simulink model "GCU_Model"  (R2018a)
settings: Solver=FixedStepDiscrete  StartTime=0.0  StopTime=1000.0  FixedStep=0.001  RelTol=1e-3  EnableMultiTasking=on
undefined symbols (not defined in the file): sigbuilder_block
libraries: simulink x1
settings Model: PacingRate=0.063000  Creator=SIMONE  LastModifiedBy=SIMONE
settings SolverCC: AutoInsertRateTranBlk=on
settings OptimizationCC: DefaultParameterBehavior=Inlined  UseFloatMulNetSlope=on  InlineInvariantSignals=on  PassReuseOutputArgsAs=Individual arguments  ZeroExternalMemoryAtStartup=off  ZeroInternalMemoryAtStartup=off  NoFixptDivByZeroProtection=on  EfficientFloat2IntCast=on  LifeSpan=1  OptimizeBlockOrder=speed  DifferentSizesBufferReuse=on
settings DebuggingCC: ParameterTunabilityLossMsg=error
settings HardwareCC: ProdBitPerPointer=32  ProdBitPerSizeT=32  ProdBitPerPtrDiffT=32  ProdLargestAtomicInteger=Long  ProdLargestAtomicFloat=Double  ProdWordSize=32  ProdLongLongMode=on  ProdHWDeviceType=ARM Compatible->ARM Cortex
settings ModelReferenceCC: ModelReferenceNumInstancesAllowed=Single
settings SFSimCC: MATLABDynamicMemAlloc=off
settings RTWCC: SystemTargetFile=ert.tlc  TemplateMakefile=ert_default_tmf  GenerateReport=on  IncludeHyperlinkInReport=on  LaunchReport=on  GenerateTraceInfo=on  GenerateTraceReport=on  GenerateTraceReportSl=on  GenerateTraceReportSf=on  GenerateTraceReportEml=on  GenerateCodeMetricsReport=on
settings CodeAppCC: ForceParamTrailComments=on  IgnoreCustomStorageClasses=off  OperatorAnnotations=on  SimulinkDataObjDesc=on  SFDataObjDesc=on  InsertBlockDesc=on
settings ERTTargetCC: TargetLangStandard=C99 (ISO)  GenerateSampleERTMain=on  IncludeMdlTerminateFcn=off  CombineSignalStateStructs=on  SupportNonFinite=off  SupportComplex=off  PurelyIntegerCode=on  SupportContinuousTime=on  SupportNonInlinedSFcns=on  InlinedParameterPlacement=NonHierarchical  ERTCustomFileTemplate=example_file_process.tlc  ERTFilePackagingFormat=CompactWithDataFile

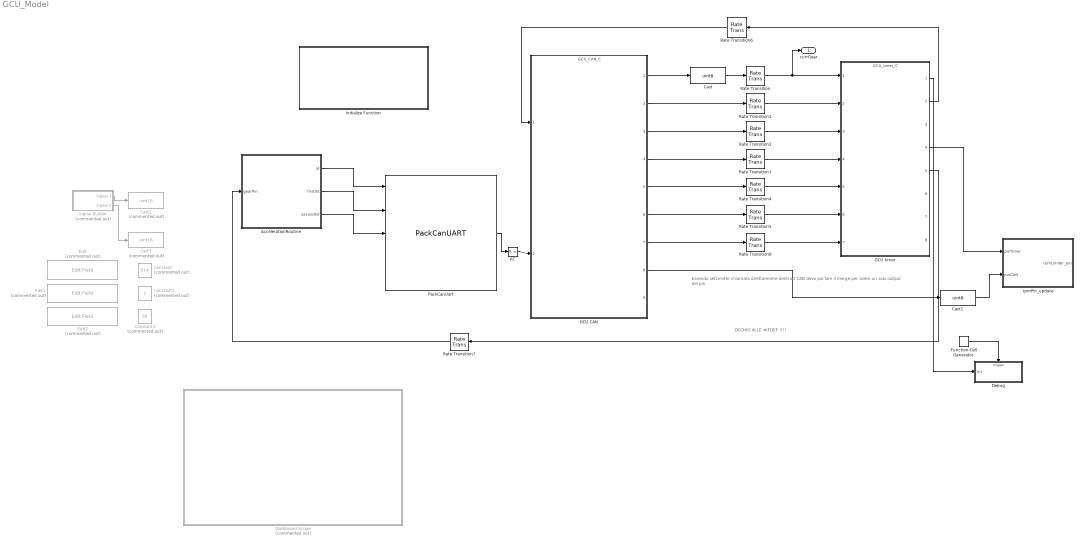
== system GCU_Model ==
  note: Essendo setLimiter chiamata direttamente dentro il CAN devo poi fare il merge
      | per avere un solo output del pin
  note: OCCHIO ALLE #IFDEF !!!!
  AccelerationRoutine : Stateflow chart  TreatAsAtomicUnit=on  SystemSampleTime=[0.01, 0.002]
  Cast : DataTypeConversion  OutDataTypeStr=uint8
  Cast1 : DataTypeConversion  OutDataTypeStr=uint8
  Cast2 : DataTypeConversion  Commented=on  OutDataTypeStr=uint16
  Cast3 : DataTypeConversion  Commented=on  OutDataTypeStr=uint16
  Constant : Constant  Commented=on  Value=514  OutDataTypeStr=uint16
  Constant2 : Constant  Commented=on  Value=2  OutDataTypeStr=uint16
  Constant3 : Constant  Commented=on  Value=30  OutDataTypeStr=uint16
  Dashboard Scope : Subsystem  Commented=on  DialogController=hmiCreateDDGDialog  IsWebBlock=on  mask(MWDashboardBlock){webBlockId=2eaf4557-9590-4f1a-91d6-635638ba46b2, webBlockType=sdiscope, ShowInitialText=on, HMISrcModelName=GCU_Model}
      mask prompts: webBlockId "WebBlock Id"; webBlockType "WebBlock Type"; HMISrcModelName "Source Model"
      mask help: SimulinkHMI:dialogs:HMIScopeDialogDesc
      mask Help: helpview([docroot '/mapfiles/simulink.map'], 'hmi_scope')
      mask Display:
      | if strcmp(get_param(bdroot(gcb),'BlockDiagramType'), 'library')
      |     image([(matlabroot) '/toolbox/simulink/hmi/icons/DashboardScope.png']);
      | end
  "Debug " : Subsystem  TreatAsAtomicUnit=on
  Edit : EditField  Commented=on  WebBlockId=100  LabelPosition=Hide  Alignment=Center
  Edit1 : EditField  Commented=on  WebBlockId=102  LabelPosition=Hide  Alignment=Center
  Edit2 : EditField  Commented=on  WebBlockId=104  LabelPosition=Hide  Alignment=Center
  Function-Call Generator : simulink/Ports & Subsystems/Function-Call Generator  sample_time=1  numberOfIterations=1
  GCU CAN : ModelReference  ModelNameDialog=GCU_CAN_C.slx  SimulationMode=Normal  ModelReferenceVersion=1.5
  GCU timer : ModelReference  ModelNameDialog=GCU_timer_C  SimulationMode=Normal  ModelReferenceVersion=1.9
  Initialize Function : Subsystem  TreatAsAtomicUnit=on
  PackCanUart : S-Function  FunctionName=PackCanUART  SFunctionDeploymentMode=off  EnableBusSupport=off
  RT : RateTransition  Deterministic=off  OutPortSampleTime=0.01
  Rate Transition{,1..8} (9 alike) : RateTransition  Deterministic=off
  Signal Builder : Subsystem  Tag=STV Subsys  Commented=on  LoadFcn=sigbuilder_block('load');  StartFcn=sigbuilder_block('start');  StopFcn=sigbuilder_block('stop');  ClipboardFcn=sigbuilder_block('clipboard');  mask(Sigbuilder block){tuvar=[0:10]}
      mask help: Simulink:masks:SigbuilderBlock_MD
      mask init:
      | if ~strcmp(get_param(bdroot(gcbh),'SimulationStatus'),'stopped') tuvar = sigbuilder_block('maskInit'); end
      settings: CopyFcn=sigbuilder_block('copy');  DeleteFcn=sigbuilder_block('delete');  ModelCloseFcn=sigbuilder_block('modelClose');  PreSaveFcn=sigbuilder_block('preSave');  PauseFcn=sigbuilder_block('pause');  ContinueFcn=sigbuilder_block('continue');  NameChangeFcn=sigbuilder_block('namechange');  OpenFcn=sigbuilder_block('open',[437.25 153 550.5 359.25 ]);  CloseFcn=sigbuilder_block('close');
      mask Display: plot(0, 0, 100, 100,[2, 2, 32, 32, 2], [68, 8, 8, 68, 68],[32, 2], [38, 38], [32, 19, 2],[53, 60, 44], [32, 17, 17, 2],[16, 16, 31, 31]);txt = getActiveGroup(gcbh);text(2, 100, txt,'verticalAlignment', 'top');
  rpmPin_update : Subsystem
  currGear : Outport
  wires:
  Signal Builder/2(Signal 2) -> Cast3/1
  Signal Builder/1(Signal 1) -> Cast2/1
  GCU CAN/1 -> Cast/1
  Rate Transition/1 -> GCU timer/1, currGear/1
  GCU CAN/2 -> Rate Transition1/1
  Rate Transition1/1 -> GCU timer/2
  GCU CAN/3 -> Rate Transition2/1
  Rate Transition2/1 -> GCU timer/3
  GCU CAN/4 -> Rate Transition3/1
  Rate Transition3/1 -> GCU timer/4
  GCU CAN/5 -> Rate Transition4/1
  Rate Transition4/1 -> GCU timer/5
  GCU CAN/6 -> Rate Transition5/1
  Rate Transition5/1 -> GCU timer/6
  GCU timer/2 -> Rate Transition6/1
  Rate Transition6/1 -> GCU CAN/1
  Cast/1 -> Rate Transition/1
  PackCanUart/1 -> RT/1
  GCU timer/5 -> Rate Transition7/1
  Rate Transition7/1 -> AccelerationRoutine/1(gearPin)
  GCU timer/4 -> rpmPin_update/1(pinTimer)
  GCU CAN/8 -> Cast1/1
  AccelerationRoutine/1(id) -> PackCanUart/1
  AccelerationRoutine/2(firstInt) -> PackCanUart/2
  AccelerationRoutine/3(secondInt) -> PackCanUart/3
  RT/1 -> GCU CAN/2
  GCU CAN/7 -> Rate Transition8/1
  Rate Transition8/1 -> GCU timer/7
  Cast1/1 -> rpmPin_update/2(pinCAN)
  Function-Call Generator/1 -> "Debug "/Trigger
  GCU timer/1 -> "Debug "/1(In1)

== system GCU_Model/Dashboard Scope ==

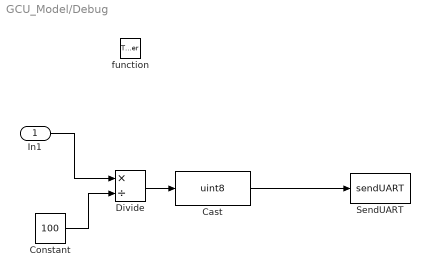
== system GCU_Model/Debug  ==
  In1 : Inport
  function : TriggerPort  TriggerType=function-call  VariantControl=Variant
  Cast : DataTypeConversion  OutDataTypeStr=uint8
  Constant : Constant  Value=100  OutDataTypeStr=uint32
  Divide : Product  Inputs=*/
  SendUART : S-Function  FunctionName=sendUART  SFunctionDeploymentMode=off  EnableBusSupport=off
  wires:
  In1/1 -> Divide/1
  Constant/1 -> Divide/2
  Divide/1 -> Cast/1
  Cast/1 -> SendUART/1

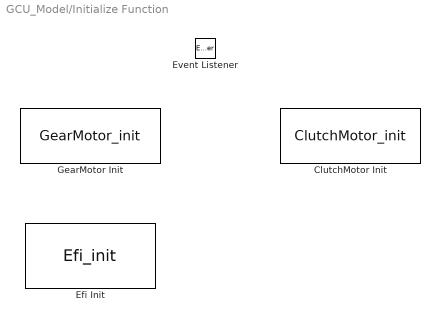
== system GCU_Model/Initialize Function ==
  ClutchMotor Init : S-Function  FunctionName=ClutchMotor_init  SFunctionDeploymentMode=off  EnableBusSupport=off
  Efi Init : S-Function  FunctionName=Efi_init  SFunctionDeploymentMode=off  EnableBusSupport=off
  Event Listener : EventListener  DisableCoverage=on  EventName=reset
  GearMotor Init : S-Function  FunctionName=GearMotor_init  SFunctionDeploymentMode=off  EnableBusSupport=off

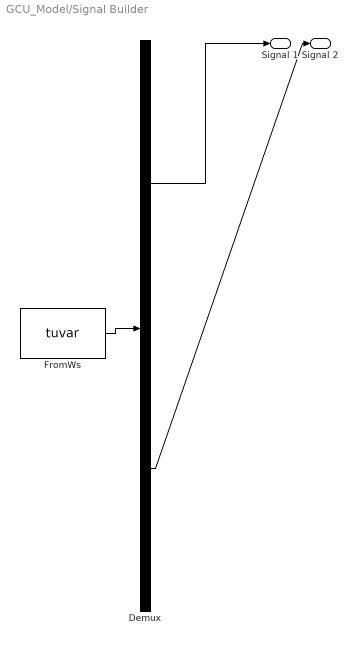
== system GCU_Model/Signal Builder ==
  Demux : Demux  Tag=STV Demux  Outputs=2
  FromWs : FromWorkspace  Tag=STV FromWs  VariableName=tuvar  SampleTime=0
      SigBuilderData=|
      | common.afterFinalStr = 'Extrapolate'
      | common.sampleTime = 0
      | dataSet.timeRange = [0 10]
      | dataSet.name = 'Group 1'
      | sbobj.Groups.Name = 'Group 1'
      | sbobj.Groups.Signals(1).Name = 'Signal 1'
      | sbobj.Groups.Signals(1).XData = [0 1 1 1.01 1.01 2 2 3 3 10]
      | sbobj.Groups.Signals(1).YData = [0 0 773 773 0 0 515 515 0 -10]
      | sbobj.Groups.Signals(2).Name = 'Signal 2'
      | sbobj.Groups.Signals(2).XData = [0 1 1 1.01 1.01 2 2 3 3 10]
      | sbobj.Groups.Signals(2).YData = [0 0 18 18 0 0 80 80 0 0]
  Signal 1 : Outport  Tag=STV Outport
  Signal 2 : Outport  Tag=STV Outport  Port=2
  wires:
  Demux/1 -> Signal 1/1
  FromWs/1 -> Demux/1
  Demux/2 -> Signal 2/1

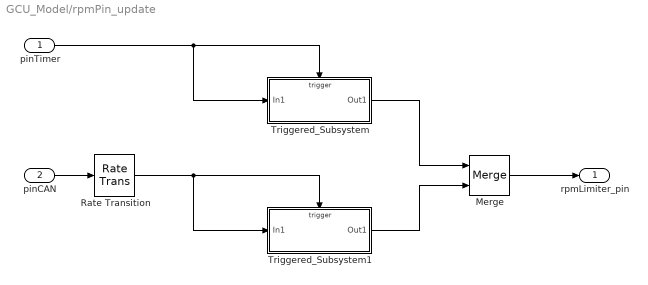
== system GCU_Model/rpmPin_update ==
  pinTimer : Inport
  pinCAN : Inport  Port=2
  Merge : Merge
  Rate Transition : RateTransition
  Triggered_Subsystem : Subsystem  TreatAsAtomicUnit=on
  Triggered_Subsystem1 : Subsystem  TreatAsAtomicUnit=on
  rpmLimiter_pin : Outport
  wires:
  pinTimer/1 -> Triggered_Subsystem/1(In1), Triggered_Subsystem/Trigger
  pinCAN/1 -> Rate Transition/1
  Triggered_Subsystem/1(Out1) -> Merge/1
  Triggered_Subsystem1/1(Out1) -> Merge/2
  Merge/1 -> rpmLimiter_pin/1
  Rate Transition/1 -> Triggered_Subsystem1/1(In1), Triggered_Subsystem1/Trigger

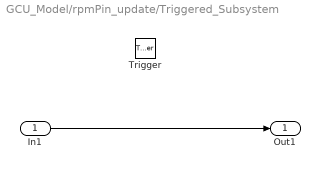
== system GCU_Model/rpmPin_update/Triggered_Subsystem ==
  In1 : Inport
  Trigger : TriggerPort  TriggerType=either  VariantControl=Variant
  Out1 : Outport
  wires:
  In1/1 -> Out1/1

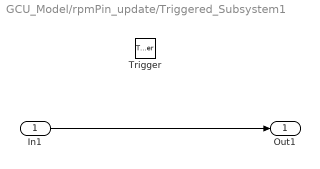
== system GCU_Model/rpmPin_update/Triggered_Subsystem1 ==
  In1 : Inport
  Trigger : TriggerPort  TriggerType=either  VariantControl=Variant
  Out1 : Outport
  wires:
  In1/1 -> Out1/1

== stateflow chart GCU_Model/AccelerationRoutine ==
  settings: executeAtInitialization=1
  state Wait
  state ActivateAac
    entry:
    %%counter =0;
    id = uint16(514);
    firstInt = uint16(1);
    %%during:counter = counter + 1;
  state InsertGear
    entry:
    id = uint16(512);
    firstInt = uint16(400);
    during:
    checkGear;
  state Ready
    id = uint16(514);
    firstInt = uint16(2);
  state EnterAcceleration
    id = uint16(1000);
    firstInt = uint16(3);
  state updateData [function]
    (default) -> (junction 20)
    (junction 20) -> (junction 24) [order 1] : [gearPin == 0 && lastGearPin == 1]
    (junction 20) -> (junction 22) [order 2]
    (junction 24) -> (junction 26) : { currGear = currGear + 1;}
    (junction 26) -> (junction 39)
    (junction 39) -> (junction 43)
    (junction 22) -> (junction 28) [order 1] : [gearPin == 1]
    (junction 22) -> (junction 30) [order 2] : {rpm = rpm + 150; wheelSpeed = wheelSpeed + 5;}
    (junction 28) -> (junction 33) : {rpm = 0; wheelSpeed = 0;}
    (junction 30) -> (junction 33) [order 1] : [message == 0]
    (junction 30) -> (junction 37) [order 2] : {message = 0; id = 774; firstInt = wheelSpeed;}
    (junction 33) -> (junction 35) : {message =1; id = 773; firstInt = currGear; secondInt = rpm;}
    (junction 37) -> (junction 35)
    (junction 35) -> (junction 43)
    (junction 43) -> (junction 46) : {lastGearPin = gearPin;}
  state DajeDeGas
    entry:
    id = uint16(0);
    rpm = uint16(0);
    wheelSpeed = uint16(0);
    during:
    updateData;
  state checkGear [function]
    (default) -> (junction 55)
    (junction 55) -> (junction 57) [order 1] : [gearPin == 0 && lastGearPin ==1]
    (junction 55) -> (junction 61) [order 2]
    (junction 57) -> (junction 59) : {currGear = currGear + 1;}
    (junction 59) -> (junction 64)
    (junction 61) -> (junction 64)
    (junction 64) -> (junction 67) : {lastGearPin = gearPin}
  state EXIT
    entry:
    id = uint16(513);
    firstInt = bitshift(uint16(100), 8);
  (default) -> Wait
  Wait -> EnterAcceleration
  InsertGear -> Ready : [currGear ==1]
  ActivateAac -> InsertGear
  EnterAcceleration -> ActivateAac
  Ready -> DajeDeGas
  DajeDeGas -> EXIT : [currGear == 5]
  data: id output uint16; firstInt output uint16; secondInt output uint16 =uint16(0);; counter local; gearPin input uint8; lastGearPin local uint8 =uint8(0); message local =0; rpm local uint16; wheelSpeed local uint16; currGear local uint16 =uint16(0);
